simulink model "tank"  (R2017b)
settings: Solver=FixedStepAuto  StartTime=0.0  StopTime=100  FixedStep=0.1  RelTol=1e-3  EnableMultiTasking=on
values from neighbouring files (symbols this model uses):
  buttomarea = calllib('tankmylib', 'buttomarea')    [RunTank.m]    (also in initialparas.mat = 1)
  heightoftank = calllib('tankmylib', 'heightoftank')    [RunTank.m]    (also in initialparas.mat = 2)
  maxinflow = calllib('tankmylib', 'maxinflow')    [RunTank.m]    (also in initialparas.mat = 0.5)
  outpipcrosssection = calllib('tankmylib', 'outpipcrosssection')    [RunTank.m]    (also in initialparas.mat = 0.05)
  overflowsensordistancefromtop = 0    [initialparas.mat]
  Timedelay = calllib('tankmylib', 'Timedelay')    [RunTank.m]    (also in initialparas.mat = 0)
settings Model: TunableVars=Timedelay,buttomarea,heightoftank,maxinflow,outpipcrosssection,overflowsensordistancefromtop  TunableVarsStorageClass=ExportedGlobal,ExportedGlobal,ExportedGlobal,ExportedGlobal,ExportedGlobal,ExportedGlobal  TunableVarsTypeQualifier=,,,,,  Creator=admin  LastModifiedBy=admin
settings DataIOCC: LimitDataPoints=on  SaveFormat=Array
settings OptimizationCC: PassReuseOutputArgsAs=Individual arguments
settings DebuggingCC: SolverPrmCheckMsg=warning  ParameterTunabilityLossMsg=error  SFUnexpectedBacktrackingDiag=warning  SFNoUnconditionalDefaultTransitionDiag=warning  SFExecutionAtInitializationDiag=none
settings HardwareCC: ProdBitPerPointer=32  ProdBitPerSizeT=32  ProdBitPerPtrDiffT=32  ProdLargestAtomicFloat=None  ProdIntDivRoundTo=Undefined  ProdEndianess=Unspecified  ProdWordSize=32  ProdHWDeviceType=32-bit Generic  TargetBitPerPointer=64  TargetBitPerSizeT=64  TargetBitPerPtrDiffT=64  TargetLongLongMode=on  TargetIntDivRoundTo=Zero  TargetEndianess=LittleEndian  TargetWordSize=64  TargetHWDeviceType=MATLAB Host  ProdEqTarget=off
settings ModelReferenceCC: PropagateSignalLabelsOutOfModel=off
settings SFSimCC: MATLABDynamicMemAlloc=off
settings RTWCC: SystemTargetFile=ert_shrlib.tlc  TemplateMakefile=ert_default_tmf  Description=Embedded Coder (host-based shared library target)  GenerateReport=on  IncludeHyperlinkInReport=on  LaunchReport=on  GenerateTraceInfo=on  GenerateTraceReport=on  GenerateTraceReportSl=on  GenerateTraceReportSf=on  GenerateTraceReportEml=on
settings CodeAppCC: ForceParamTrailComments=on  IgnoreCustomStorageClasses=off  OperatorAnnotations=on  SimulinkDataObjDesc=on  SFDataObjDesc=on  MATLABFcnDesc=on  InsertBlockDesc=on  StateflowObjectComments=on  MATLABSourceComments=on
settings STFCustomTargetCC: MultiwordLength=256  GenerateSampleERTMain=on  ParMdlRefBuildCompliant=on  CompOptLevelCompliant=on  CombineOutputUpdateFcns=on  ERTCustomFileBanners=on  SupportComplex=off  SupportNonInlinedSFcns=off  RemoveResetFunc=on  MATLABClassNameForMDSCustomization=Simulink.SoftwareTarget.ERTCustomization  ModelStepFunctionPrototypeControlCompliant=on  GRTInterface=off  UseToolchainInfoCompliant=on  SystemTargetFile=ert_shrlib.tlc
settings ERTTargetCC: GenerateSampleERTMain=on  ConcurrentExecutionCompliant=off  SupportComplex=off  SupportContinuousTime=on  CPPClassGenCompliant=off  ERTCustomFileTemplate=example_file_process.tlc
settings ConfigComp: CovMetricSettings=dw  CovHtmlReporting=on  CovSaveCumulativeToWorkspaceVar=on  CovSaveSingleToWorkspaceVar=on  CovExternalEMLEnable=off  CovSFcnEnable=off

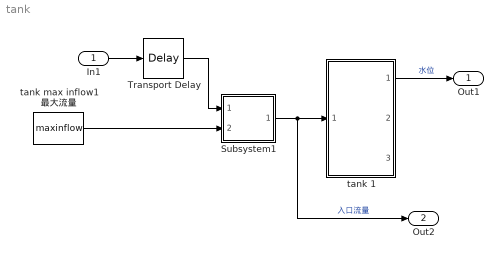
== system tank ==
  In1 : Inport
  Subsystem1 : Subsystem  mask(Valve){InitialPosition=0}
      mask prompts: InitialPosition "Initial position [0=closed 1=open]:"
      mask help: Valve
      mask Display: disp('VALVE')
  Transport Delay : TransportDelay  DelayTime=Timedelay
  tank 1 : Subsystem  mask(Water tank){ht=heightoftank, area=buttomarea, outletArea=outpipcrosssection, overflowLimit=overflowsensordistancefromtop, initialHt=0.5}
      mask prompts: ht "Height of tank (m):"; area "Bottom area (m^2):"; outletArea "Out pipe crossection (m^2):"; overflowLimit "Overflow sensor distance from top (m):"; initialHt "Initial level height (m):"
      mask help: Cylindrical water tank with overflow signal
      mask Display: disp('WATER\nTANK')
  tank max inflow1 最大流量 : Constant  Value=maxinflow
  Out1 : Outport
  Out2 : Outport  Port=2
  wires:
  tank max inflow1 最大流量/1 -> Subsystem1/2(source flow)
  Subsystem1/1(out flow) -> Out2/1, tank 1/1(flow in)  "入口流量"
  In1/1 -> Transport Delay/1
  tank 1/1(water level) -> Out1/1  "水位"
  Transport Delay/1 -> Subsystem1/1(control)

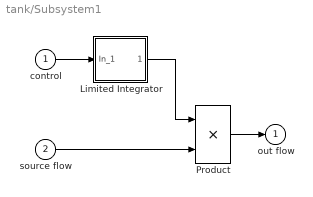
== system tank/Subsystem1 ==
  control : Inport
  source flow : Inport  Port=2
  Limited Integrator : Subsystem  mask(Limited integrator.){lb=0, ub=1, xi=InitialPosition}
      mask prompts: lb "Lower bound:"; ub "Upper bound:"; xi "Initial condition"
      mask help: Limited integrator
      mask Help: Implements a limited integrator with \nan expression of the form:\n\nif(x<=lb and u<0) or (x>=ub and u>0)\n\txdot=0\nelse\n\txdot=u.
      mask Display: plot(-1,-0.2,3.5,1.2,[0.05,1,2,2.9],[0,0,1,1]);disp(' 1/s    ')
  Product : Product  SaturateOnIntegerOverflow=on  RndMeth=Zero  InputSameDT=on  OutDataTypeStr=Inherit: Same as first input
  out flow : Outport  InitialOutput=0
  wires:
  source flow/1 -> Product/2
  Product/1 -> out flow/1
  control/1 -> Limited Integrator/1(In_1)
  Limited Integrator/1(Out_1) -> Product/1

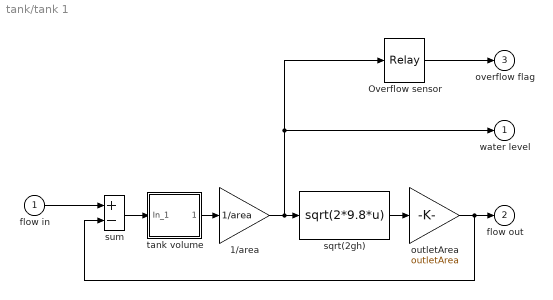
== system tank/tank 1 ==
  flow in : Inport
  1/area : Gain  Gain=1/area  SaturateOnIntegerOverflow=on  OutDataTypeStr=Inherit: Same as input  ParamDataTypeStr=Inherit: Same as input
  Overflow sensor : Relay  OnSwitchValue=ht - overflowLimit  OffSwitchValue=ht - overflowLimit
  outletArea : Gain  Gain=outletArea  SaturateOnIntegerOverflow=on  OutDataTypeStr=Inherit: Same as input  ParamDataTypeStr=Inherit: Same as input
  sqrt(2gh) : Fcn  Expr=sqrt(2*9.8*u)
  sum : Sum  Inputs=+-  SaturateOnIntegerOverflow=on  InputSameDT=on  OutDataTypeStr=Inherit: Same as first input
  tank volume : Subsystem  mask(Limited integrator.){lb=0, ub=ht * area, xi=initialHt * area}
      mask prompts: lb "Lower bound:"; ub "Upper bound:"; xi "Initial condition"
      mask help: Limited integrator
      mask Help: Implements a limited integrator with \nan expression of the form:\n\nif(x<=lb and u<0) or (x>=ub and u>0)\n\txdot=0\nelse\n\txdot=u.
      mask Display: plot(-1,-0.2,3.5,1.2,[0.05,1,2,2.9],[0,0,1,1]);disp(' 1/s    ')
  water level : Outport  InitialOutput=0
  flow out : Outport  Port=2  InitialOutput=0
  overflow flag : Outport  Port=3  InitialOutput=0
  wires:
  outletArea/1 -> flow out/1, sum/2
  sqrt(2gh)/1 -> outletArea/1
  1/area/1 -> Overflow sensor/1, water level/1, sqrt(2gh)/1
  tank volume/1(Out_1) -> 1/area/1
  Overflow sensor/1 -> overflow flag/1
  flow in/1 -> sum/1
  sum/1 -> tank volume/1(In_1)

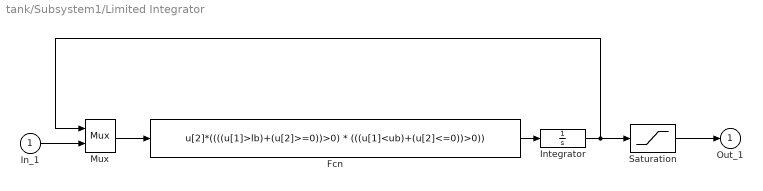
== system tank/Subsystem1/Limited Integrator ==
  In_1 : Inport
  Fcn : Fcn  Expr=u[2]*((((u[1]>lb)+(u[2]>=0))>0) * (((u[1]<ub)+(u[2]<=0))>0))
  Integrator : Integrator  InitialCondition=xi
  Mux : Mux  Inputs=2
  Saturation : Saturate  UpperLimit=ub  LowerLimit=lb
  Out_1 : Outport  InitialOutput=0
  wires:
  Integrator/1 -> Saturation/1, Mux/1
  Fcn/1 -> Integrator/1
  Mux/1 -> Fcn/1
  In_1/1 -> Mux/2
  Saturation/1 -> Out_1/1

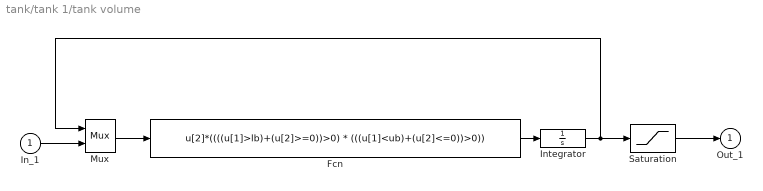
== system tank/tank 1/tank volume ==
  In_1 : Inport
  Fcn : Fcn  Expr=u[2]*((((u[1]>lb)+(u[2]>=0))>0) * (((u[1]<ub)+(u[2]<=0))>0))
  Integrator : Integrator  InitialCondition=xi
  Mux : Mux  Inputs=2
  Saturation : Saturate  UpperLimit=ub  LowerLimit=lb
  Out_1 : Outport  InitialOutput=0
  wires:
  Integrator/1 -> Saturation/1, Mux/1
  Fcn/1 -> Integrator/1
  Mux/1 -> Fcn/1
  In_1/1 -> Mux/2
  Saturation/1 -> Out_1/1
